simulink model "F28379D_benchTest_demo1_CPU1"  (R2019b)
settings: Solver=FixedStepDiscrete  StartTime=0.0  StopTime=Inf  RelTol=1e-3  EnableMultiTasking=on
PreLoadFcn:
  | RTWConfigurationCB('preloadfcn', bdroot);
undefined symbols (not defined in the file or in its folder): Down, GPTRIP1SEL, GPTRIP2SEL, LEDPWM, TZ1, TZ2, Up
libraries: c280xlib x3, simulink x3, c2837xDlib x3, c2802xlib x2, canmsglib x1, hdlsllib x1
settings Model: DataDictionary=F28379D_benchTest_demo1.sldd  ExtModeTrigDuration=8  Creator=Nick  LastModifiedBy=Nick
settings OptimizationCC: DefaultUnderspecifiedDataType=single  EnhancedBackFolding=on  PassReuseOutputArgsAs=Individual arguments  MaxStackSize=1024  OptimizeBlockOrder=speed  DifferentSizesBufferReuse=on  OptimizationCustomize=off  DenormalBehavior=FlushToZero  EfficientTunableParamExpr=on
settings DebuggingCC: ParameterTunabilityLossMsg=error
settings HardwareCC: ProdBitPerChar=16  ProdBitPerInt=16  ProdBitPerPointer=32  ProdBitPerSizeT=32  ProdBitPerPtrDiffT=32  ProdLargestAtomicInteger=Integer  ProdLargestAtomicFloat=None  ProdWordSize=16  ProdLongLongMode=on  ProdHWDeviceType=Texas Instruments->C2000
settings SFSimCC: MATLABDynamicMemAlloc=off
settings RTWCC: SystemTargetFile=ert.tlc  HardwareBoard=TI Delfino F28379D LaunchPad  TLCOptions=-aInlineSetEventsForThisBaseRateFcn=TLC_FALSE -aSuppressMultiTaskScheduler=TLC_FALSE -aRateBasedStepFcn=1  TemplateMakefile=ert_default_tmf  GenerateReport=on  Toolchain=Texas Instruments Code Composer Studio (C2000)  IncludeHyperlinkInReport=on  LaunchReport=on  GenerateTraceInfo=on  GenerateTraceReport=on  GenerateTraceReportSl=on  GenerateTraceReportSf=on  GenerateTraceReportEml=on
settings CodeAppCC: ForceParamTrailComments=on  IgnoreCustomStorageClasses=off  OperatorAnnotations=on  SimulinkDataObjDesc=on  SFDataObjDesc=on  InsertBlockDesc=on
settings ERTTargetCC: CodeReplacementLibrary=TI C28x  GenerateASAP2=on  ExtModeStaticAllocSize=10000

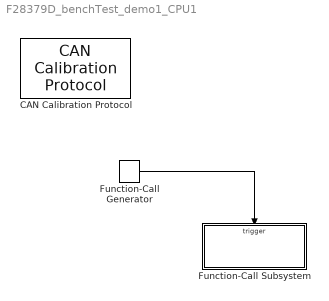
== system F28379D_benchTest_demo1_CPU1 ==
  CAN Calibration Protocol : c280xlib/CAN Calibration Protocol  CCP_STATION_ID=hex2dec('1')  module=eCAN_B  ccp_cro_id=hex2dec('6FA')  ccp_cro_message_type=Standard (11-bit identifier)  ccp_return_id=hex2dec('6FB')  ccp_return_message_type=Standard (11-bit identifier)  TOTAL_NUM_ODTS=20  cro_sample_time=0.1
      settings: SourceProductName=Embedded Coder Support Package for Texas Instruments C2000 Processors  SourceProductBaseCode=TIC2000
  Function-Call Generator : simulink/Ports & Subsystems/Function-Call Generator  sample_time=.001  numberOfIterations=1
  Function-Call Subsystem : Subsystem  TreatAsAtomicUnit=on
  wires:
  Function-Call Generator/1 -> Function-Call Subsystem/Trigger

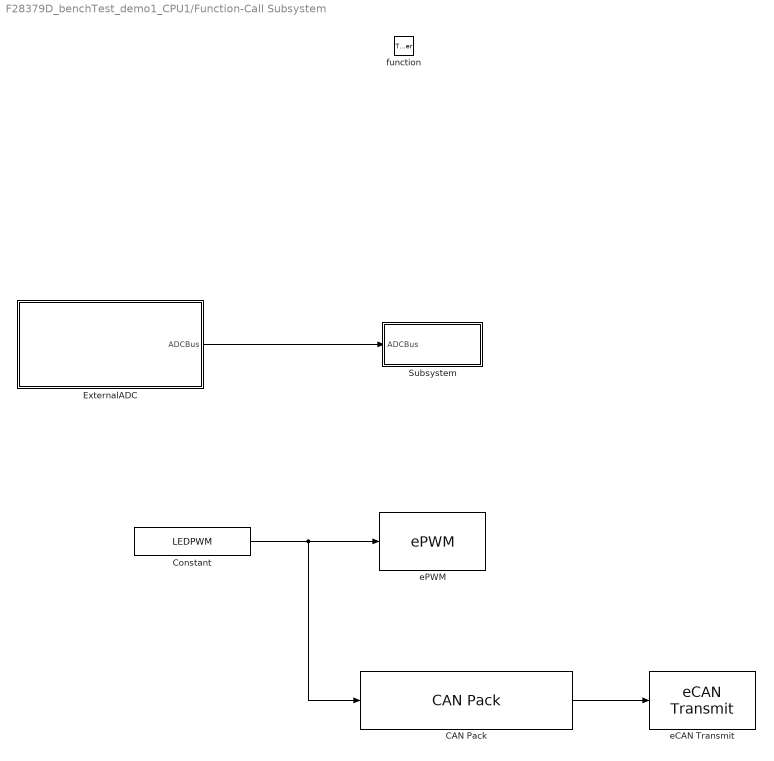
== system F28379D_benchTest_demo1_CPU1/Function-Call Subsystem ==
  function : TriggerPort  TriggerType=function-call  VariantControl=Variant
  CAN Pack : canmsglib/CAN Pack  MsgList=(none)  MsgName=CAN Msg  MsgIDType=Standard (11-bit identifier)  MsgIdentifier=10  MsgLength=8  Remote=off  ApplyMinMax=off  BusOutput=off  SignalInfo={ 'PWM', '0', '16', 'LE', 'signed', 'Standard', '0', '1', '0', '-Inf', 'Inf' }
      settings: SourceProductName=Vehicle Network Toolbox  SourceProductBaseCode=VN  DataFormat=manually specified signals
  Constant : Constant  Value=LEDPWM  SampleTime=-1
  ExternalADC : Subsystem
  Subsystem : Subsystem
  eCAN Transmit : c280xlib/eCAN Transmit  chipFamily=C280x  useModule=eCAN_B  mailboxNo=3  messageID=bin2dec('111000111')  messageType=Standard (11-bit identifier)  enableBlockingMode=off  postInterrupt=off  interruptLine=0
      settings: SourceProductName=Embedded Coder Support Package for Texas Instruments C2000 Processors  SourceProductBaseCode=TIC2000
  ePWM : c2802xlib/ePWM  useModule=ePWM12  ePWMxLINKTBPRD=Not Linked  periodUnits=Seconds  timerSource=Specify via dialog  timerPeriod_clk=64000  timerPeriod_sec=0.0001  tbshadow=Counter equals to zero  countingMode=Up-Down  phaseActiveEnable=Disable  phaseDirection=Count down after sync  phaseActive=0  synchronizationEnable=off  dcaevt1Sync=off  dcbevt1Sync=off  synchronizationOption=Disable  clockPrescale=1  HSclockPrescale=1  enswap=off  ePWMxAStatus=on  ePWMxAactionLogic1=Set  ePWMxAactionLogic2=Clear  ePWMxAactionLogic3=Clear  ePWMxAactionLogic4=Set  ePWMxAactionLogic5=Do nothing  ePWMxAactionLogic6=Do nothing  ePWMxALoadMode=Load on counter equals to zero (CTR=Zero)  ePWMxACSFenable=off  ePWMxACSFvalue=Forcing disable  ePWMxASFreload=Zero  ePWMxBStatus=off  ePWMxBactionLogic1=Set  ePWMxBactionLogic2=Clear  ePWMxBactionLogic3=Do nothing  ePWMxBactionLogic4=Do nothing  ePWMxBactionLogic5=Clear  ePWMxBactionLogic6=Set  ePWMxBLoadMode=Load on counter equals to zero (CTR=Zero)  ePWMxBCSFenable=off  ePWMxBCSFvalue=Forcing disable  ePWMxBSFreload=Zero  ePWNxBOutWay=off  ePWMxLINKCMPA=Not Linked  CMPAUnits=Percentages  CMPASource=Input port  CMPAValue_per=0  CMPAValue_clk=32000  enCMPAshadow=Counter equals to zero  ePWMxLINKCMPB=Not Linked  CMPBUnits=Clock cycles  CMPBSource=Specify via dialog  CMPBValue_per=50  CMPBValue_clk=32000  enCMPBshadow=Counter equals to zero  ePWMxLINKCMPC=Not Linked  CMPCUnits=Clock cycles  CMPCSource=Specify via dialog  CMPCValue_per=50  CMPCValue_clk=32000  enCMPCshadow=Counter equals to zero  ePWMxLINKCMPD=Not Linked  CMPDUnits=Clock cycles  CMPDSource=Specify via dialog  CMPDValue_per=50  CMPDValue_clk=32000  enCMPDshadow=Counter equals to zero  enableDBePWMxA=off  enableDBePWMxB=off  enhalfcycle=off  DBpolarity=Active high (AH)  DBedgeDelay=Positive  DBSource_ePWMxA=ePWMxA  DBSource_ePWMxB=ePWMxA  DBperiodSource=Specify via dialog  REDperiod=0  FEDperiod=0  adcstartModuleA=off  adcrequestEventA=First event  adcstartEventA=Digital Compare Module A Event 1 start of conversion (DCAEVT1.soc)  adcstartEventA_type2=Digital Compare Module A Event 1 start of conversion (DCAEVT1.soc)  adcstartModuleB=off  adcrequestEventB=First event  adcstartEventB=Counter equals to zero (CTR=Zero)  adcstartEventB_type2=Counter equals to zero (CTR=Zero)  intEn=off  intPrd=First event  intSel=Counter equals to zero (CTR=Zero)  intSel_type2=Counter equals to zero (CTR=Zero)  hrpe=off  enHRPWM=off  HRPWM_LoadMode=Counter equals to period (CTR=PRD)  HRPWM_CTLMode=Duty or Period control mode  HRPWM_EDGMode=Both edge  hrpeb=off  enHRPWMB=off  HRPWM_LoadModeB=Counter equals to zero (CTR=ZERO)  HRPWM_CTLModeB=Duty or Period control mode  HRPWM_EDGModeB=Both edge  enSFO=on  enautoconv=on  chopperEnable=off  chopperFrequency=1  chopperFirstwidth=1  chopperDuty=12.5%  tripZonesource=Specify via dialog  tzselOSHT1=off  tzselOSHT2=off  tzselOSHT3=off  tzselOSHDCAEV1=off  tzselOSHDCBEV1=off  tzselCBC1=off  tzselCBC2=off  tzselCBC3=off  tzselCBCDCAEV2=off  tzselCBCDCBEV2=off  tzselOSHT4=off  tzselOSHT5=off  tzselOSHT6=off  tzselCBC4=off  tzselCBC5=off  tzselCBC6=off  enTzOstIntr=off  enTzCbcIntr=off  enTzDCAEVT1Intr=off  enTzDCAEVT2Intr=off  enTzDCBEVT1Intr=off  enTzDCBEVT2Intr=off  ePWMxAforced=No action  ePWMxBforced=No action  DCAEVT1forced=No action  DCBEVT1forced=No action  DCAEVT2forced=No action  DCBEVT2forced=No action  dcah=Trip Zone 1 input (TZ1)  dcal=Trip Zone 2 input (TZ2)  dcbh=Trip Zone 1 input (TZ1)  dcbl=Trip Zone 2 input (TZ2)  dcah_type2=GPTRIP1SEL/(TZ1)  dcal_type2=GPTRIP2SEL/(TZ2)  dcbh_type2=GPTRIP1SEL/(TZ1)  dcbl_type2=GPTRIP2SEL/(TZ2)  gendcaevt1=Event disabled  gendcaevt2=Event disabled  gendcbevt1=Event disabled  gendcbevt2=Event disabled  dcaevt1src=DCAEVT1 with sync  dcaevt2src=DCAEVT2 with sync  dcbevt1src=DCBEVT1 with sync  dcbevt2src=DCBEVT2 with sync  pulsesel=Counter equals to zero (CTR=Zero)  blankinv=off  blankoffset=0  blankwidth=0  evsrcsel=Filtered version of DCAEVT1 (DCAEVT1FILT)  encape=off  PwmType=C2000_Type4
      settings: SourceProductName=Embedded Coder Support Package for Texas Instruments C2000 Processors
  wires:
  ExternalADC/1(ADCBus) -> Subsystem/1(ADCBus)
  Constant/1 -> CAN Pack/1, ePWM/1
  CAN Pack/1 -> eCAN Transmit/1

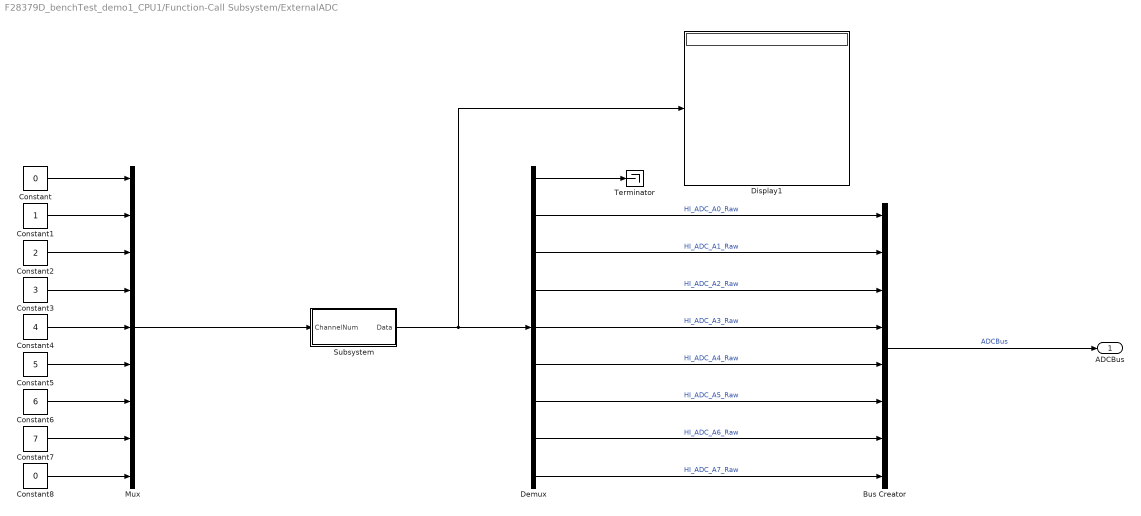
== system F28379D_benchTest_demo1_CPU1/Function-Call Subsystem/ExternalADC ==
  Bus Creator : BusCreator  Inputs=8
  Constant : Constant  Value=0
  Constant1 : Constant
  Constant2 : Constant  Value=2
  Constant3 : Constant  Value=3
  Constant4 : Constant  Value=4
  Constant5 : Constant  Value=5
  Constant6 : Constant  Value=6
  Constant7 : Constant  Value=7
  Constant8 : Constant  Value=0
  Demux : Demux  Outputs=9
  Display1 : Display
  Mux : Mux  Inputs=9
  Subsystem : Subsystem
  Terminator : Terminator
  ADCBus : Outport
  wires:
  Constant6/1 -> Mux/7
  Demux/1 -> Terminator/1
  Constant7/1 -> Mux/8
  Mux/1 -> Subsystem/1(ChannelNum)
  Demux/5 -> Bus Creator/4  "HI_ADC_A3_Raw"
  Constant8/1 -> Mux/9
  Demux/2 -> Bus Creator/1  "HI_ADC_A0_Raw"
  Constant2/1 -> Mux/3
  Demux/8 -> Bus Creator/7  "HI_ADC_A6_Raw"
  Demux/7 -> Bus Creator/6  "HI_ADC_A5_Raw"
  Constant5/1 -> Mux/6
  Constant/1 -> Mux/1
  Constant4/1 -> Mux/5
  Bus Creator/1 -> ADCBus/1  "ADCBus"
  Demux/3 -> Bus Creator/2  "HI_ADC_A1_Raw"
  Demux/9 -> Bus Creator/8  "HI_ADC_A7_Raw"
  Demux/4 -> Bus Creator/3  "HI_ADC_A2_Raw"
  Constant1/1 -> Mux/2
  Constant3/1 -> Mux/4
  Demux/6 -> Bus Creator/5  "HI_ADC_A4_Raw"
  Subsystem/1(Data) -> Display1/1, Demux/1

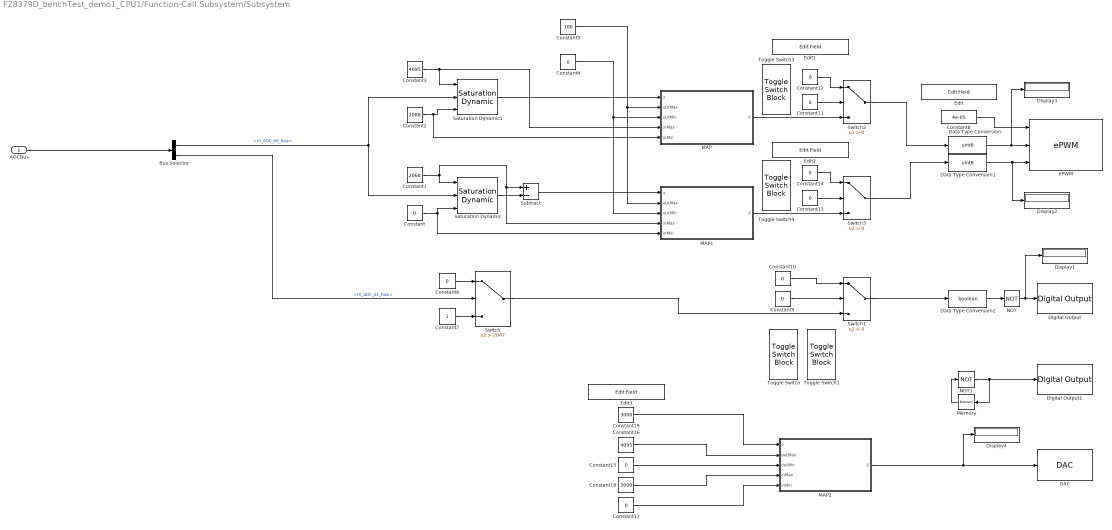
== system F28379D_benchTest_demo1_CPU1/Function-Call Subsystem/Subsystem ==
  ADCBus : Inport
  Bus Selector : BusSelector  OutputSignals=HI_ADC_A0_Raw,HI_ADC_A1_Raw
  Constant{,4,6,9..15,17} (11 alike) : Constant  Value=0
  Constant1 : Constant  Value=2068
  Constant16 : Constant  Value=4095
  Constant18 : Constant  Value=3000
  Constant19 : Constant  Value=3000
  Constant2 : Constant  Value=2088
  Constant3 : Constant  Value=4095
  Constant5 : Constant  Value=100
  Constant7 : Constant
  Constant8 : Constant  Value=4e-05
  DAC : c2837xDlib/DAC  channel=A  saturate=on
      settings: SourceProductName=Embedded Coder Support Package for Texas Instruments C2000 Processors  SourceProductBaseCode=TIC2000
  Data Type Conversion : DataTypeConversion  OutDataTypeStr=uint8
  Data Type Conversion1 : DataTypeConversion  OutDataTypeStr=uint8
  Data Type Conversion2 : DataTypeConversion  OutDataTypeStr=boolean
  Digital Output : c2837xDlib/Digital Output  GPIO_Number=GPIO16~GPIO23  GPIO_Bit0=on  GPIO_BIT0_Toggle=off  GPIO_Bit1=off  GPIO_BIT1_Toggle=off  GPIO_Bit2=off  GPIO_BIT2_Toggle=off  GPIO_Bit3=off  GPIO_BIT3_Toggle=off  GPIO_Bit4=off  GPIO_BIT4_Toggle=off  GPIO_Bit5=off  GPIO_BIT5_Toggle=off  GPIO_Bit6=off  GPIO_BIT6_Toggle=off  GPIO_Bit7=off  GPIO_BIT7_Toggle=off
      settings: SourceProductName=Embedded Coder Support Package for Texas Instruments C2000 Processors  SourceProductBaseCode=TIC2000
  Digital Output1 : c2837xDlib/Digital Output  GPIO_Number=GPIO64~GPIO71  GPIO_Bit0=off  GPIO_BIT0_Toggle=off  GPIO_Bit1=off  GPIO_BIT1_Toggle=off  GPIO_Bit2=off  GPIO_BIT2_Toggle=off  GPIO_Bit3=on  GPIO_BIT3_Toggle=off  GPIO_Bit4=off  GPIO_BIT4_Toggle=off  GPIO_Bit5=off  GPIO_BIT5_Toggle=off  GPIO_Bit6=off  GPIO_BIT6_Toggle=off  GPIO_Bit7=off  GPIO_BIT7_Toggle=off
      settings: SourceProductName=Embedded Coder Support Package for Texas Instruments C2000 Processors  SourceProductBaseCode=TIC2000
  Display{1..4} (4 alike) : Display
  Edit{,1..3} (4 alike) : EditField  LabelPosition=Hide  ShowInitialText=on  Alignment=Center
  MAP : Subsystem
  MAP1 : Subsystem
  MAP2 : Subsystem
  Memory : Memory  InheritSampleTime=on
  NOT : Logic  Operator=NOT  IconShape=distinctive  AllPortsSameDT=off  OutDataTypeStr=boolean
  NOT1 : Logic  Operator=NOT  IconShape=distinctive  AllPortsSameDT=off  OutDataTypeStr=boolean
  Saturation Dynamic : simulink/Discontinuities/Saturation Dynamic  OutMin=[]  OutMax=[]  OutDataTypeStr=Inherit: Same as second input  OutDataType=fixdt(1, 16)  OutScaling=2^-10  DoSatur=off
  Saturation Dynamic1 : simulink/Discontinuities/Saturation Dynamic  OutMin=[]  OutMax=[]  OutDataTypeStr=Inherit: Same as second input  OutDataType=fixdt(1, 16)  OutScaling=2^-10  DoSatur=off
  Subtract : Sum  Inputs=+-
  Switch : Switch  Criteria=u2 > Threshold  Threshold=2047
  Switch1 : Switch  Criteria=u2 > Threshold
  Switch2 : Switch  Criteria=u2 > Threshold
  Switch3 : Switch  Criteria=u2 > Threshold
  Toggle Switch{,1,3..4} (4 alike) : ToggleSwitchBlock
  ePWM : c2802xlib/ePWM  useModule=ePWM2  ePWMxLINKTBPRD=Not Linked  periodUnits=Seconds  timerSource=Input port  timerPeriod_clk=64000  timerPeriod_sec=0.0001  tbshadow=Counter equals to zero  countingMode=Up-Down  phaseActiveEnable=Disable  phaseDirection=Count down after sync  phaseActive=0  synchronizationEnable=off  dcaevt1Sync=off  dcbevt1Sync=off  synchronizationOption=Disable  clockPrescale=1  HSclockPrescale=1  enswap=off  ePWMxAStatus=on  ePWMxAactionLogic1=Set  ePWMxAactionLogic2=Clear  ePWMxAactionLogic3=Clear  ePWMxAactionLogic4=Set  ePWMxAactionLogic5=Do nothing  ePWMxAactionLogic6=Do nothing  ePWMxALoadMode=Load on counter equals to zero (CTR=Zero)  ePWMxACSFenable=off  ePWMxACSFvalue=Forcing disable  ePWMxASFreload=Zero  ePWMxBStatus=on  ePWMxBactionLogic1=Set  ePWMxBactionLogic2=Clear  ePWMxBactionLogic3=Do nothing  ePWMxBactionLogic4=Do nothing  ePWMxBactionLogic5=Clear  ePWMxBactionLogic6=Set  ePWMxBLoadMode=Load on counter equals to zero (CTR=Zero)  ePWMxBCSFenable=off  ePWMxBCSFvalue=Forcing disable  ePWMxBSFreload=Zero  ePWNxBOutWay=off  ePWMxLINKCMPA=Not Linked  CMPAUnits=Percentages  CMPASource=Input port  CMPAValue_per=0  CMPAValue_clk=32000  enCMPAshadow=Counter equals to zero  ePWMxLINKCMPB=Not Linked  CMPBUnits=Percentages  CMPBSource=Input port  CMPBValue_per=0  CMPBValue_clk=32000  enCMPBshadow=Counter equals to zero  ePWMxLINKCMPC=Not Linked  CMPCUnits=Clock cycles  CMPCSource=Specify via dialog  CMPCValue_per=50  CMPCValue_clk=32000  enCMPCshadow=Counter equals to zero  ePWMxLINKCMPD=Not Linked  CMPDUnits=Clock cycles  CMPDSource=Specify via dialog  CMPDValue_per=50  CMPDValue_clk=32000  enCMPDshadow=Counter equals to zero  enableDBePWMxA=off  enableDBePWMxB=off  enhalfcycle=off  DBpolarity=Active high (AH)  DBedgeDelay=Positive  DBSource_ePWMxA=ePWMxA  DBSource_ePWMxB=ePWMxA  DBperiodSource=Specify via dialog  REDperiod=0  FEDperiod=0  adcstartModuleA=off  adcrequestEventA=First event  adcstartEventA=Digital Compare Module A Event 1 start of conversion (DCAEVT1.soc)  adcstartEventA_type2=Digital Compare Module A Event 1 start of conversion (DCAEVT1.soc)  adcstartModuleB=off  adcrequestEventB=First event  adcstartEventB=Counter equals to zero (CTR=Zero)  adcstartEventB_type2=Counter equals to zero (CTR=Zero)  intEn=off  intPrd=First event  intSel=Counter equals to zero (CTR=Zero)  intSel_type2=Counter equals to zero (CTR=Zero)  hrpe=off  enHRPWM=off  HRPWM_LoadMode=Counter equals to period (CTR=PRD)  HRPWM_CTLMode=Duty or Period control mode  HRPWM_EDGMode=Both edge  hrpeb=off  enHRPWMB=off  HRPWM_LoadModeB=Counter equals to zero (CTR=ZERO)  HRPWM_CTLModeB=Duty or Period control mode  HRPWM_EDGModeB=Both edge  enSFO=on  enautoconv=on  chopperEnable=off  chopperFrequency=1  chopperFirstwidth=1  chopperDuty=12.5%  tripZonesource=Specify via dialog  tzselOSHT1=off  tzselOSHT2=off  tzselOSHT3=off  tzselOSHDCAEV1=off  tzselOSHDCBEV1=off  tzselCBC1=off  tzselCBC2=off  tzselCBC3=off  tzselCBCDCAEV2=off  tzselCBCDCBEV2=off  tzselOSHT4=off  tzselOSHT5=off  tzselOSHT6=off  tzselCBC4=off  tzselCBC5=off  tzselCBC6=off  enTzOstIntr=off  enTzCbcIntr=off  enTzDCAEVT1Intr=off  enTzDCAEVT2Intr=off  enTzDCBEVT1Intr=off  enTzDCBEVT2Intr=off  ePWMxAforced=No action  ePWMxBforced=No action  DCAEVT1forced=No action  DCBEVT1forced=No action  DCAEVT2forced=No action  DCBEVT2forced=No action  dcah=Trip Zone 1 input (TZ1)  dcal=Trip Zone 2 input (TZ2)  dcbh=Trip Zone 1 input (TZ1)  dcbl=Trip Zone 2 input (TZ2)  dcah_type2=GPTRIP1SEL/(TZ1)  dcal_type2=GPTRIP2SEL/(TZ2)  dcbh_type2=GPTRIP1SEL/(TZ1)  dcbl_type2=GPTRIP2SEL/(TZ2)  gendcaevt1=Event disabled  gendcaevt2=Event disabled  gendcbevt1=Event disabled  gendcbevt2=Event disabled  dcaevt1src=DCAEVT1 with sync  dcaevt2src=DCAEVT2 with sync  dcbevt1src=DCBEVT1 with sync  dcbevt2src=DCBEVT2 with sync  pulsesel=Counter equals to zero (CTR=Zero)  blankinv=off  blankoffset=0  blankwidth=0  evsrcsel=Filtered version of DCAEVT1 (DCAEVT1FILT)  encape=off  PwmType=C2000_Type4
      settings: SourceProductName=Embedded Coder Support Package for Texas Instruments C2000 Processors
  wires:
  ADCBus/1 -> Bus Selector/1
  Bus Selector/1 -> Saturation Dynamic/2, Saturation Dynamic1/2  "<HI_ADC_A0_Raw>"
  Constant/1 -> MAP1/5(inMin), Saturation Dynamic/3
  Constant1/1 -> Subtract/1, MAP1/4(inMax), Saturation Dynamic/1
  Subtract/1 -> MAP1/1(x)
  Constant3/1 -> Saturation Dynamic1/1, MAP/4(inMax)
  Constant2/1 -> MAP/5(inMin), Saturation Dynamic1/3
  Saturation Dynamic1/1 -> MAP/1(x)
  Constant4/1 -> MAP1/3(outMin), MAP/3(outMin)
  Constant5/1 -> MAP1/2(outMax), MAP/2(outMax)
  MAP/1(X) -> Switch2/3
  Saturation Dynamic/1 -> Subtract/2
  Switch/1 -> Switch1/3
  Bus Selector/2 -> Switch/2  "<HI_ADC_A1_Raw>"
  Constant6/1 -> Switch/1
  Constant7/1 -> Switch/3
  Data Type Conversion/1 -> Display3/1, ePWM/2
  Data Type Conversion1/1 -> Display2/1, ePWM/3
  Constant8/1 -> ePWM/1
  Data Type Conversion2/1 -> NOT/1
  NOT/1 -> Display1/1, Digital Output/1
  Switch1/1 -> Data Type Conversion2/1
  Constant9/1 -> Switch1/2
  Constant10/1 -> Switch1/1
  Switch2/1 -> Data Type Conversion/1
  Constant11/1 -> Switch2/2
  Constant12/1 -> Switch2/1
  Switch3/1 -> Data Type Conversion1/1
  MAP1/1(X) -> Switch3/3
  Constant13/1 -> Switch3/2
  Constant14/1 -> Switch3/1
  Memory/1 -> NOT1/1
  NOT1/1 -> Memory/1, Digital Output1/1
  MAP2/1(X) -> Display4/1, DAC/1
  Constant16/1 -> MAP2/2(outMax)
  Constant15/1 -> MAP2/3(outMin)
  Constant18/1 -> MAP2/4(inMax)
  Constant17/1 -> MAP2/5(inMin)
  Constant19/1 -> MAP2/1(x)

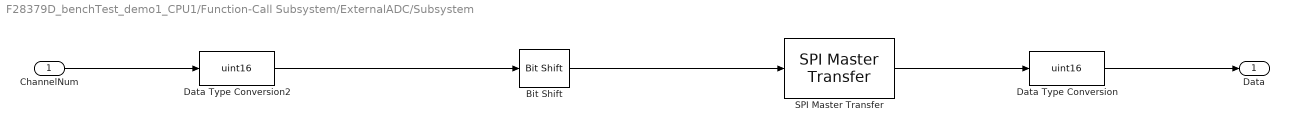
== system F28379D_benchTest_demo1_CPU1/Function-Call Subsystem/ExternalADC/Subsystem ==
  ChannelNum : Inport
  Bit Shift : hdlsllib/Logic and Bit Operations/Bit Shift  mode=Shift Left Logical  N=11
      settings: SourceProductName=Simulink
  Data Type Conversion : DataTypeConversion  OutDataTypeStr=uint16
  Data Type Conversion2 : DataTypeConversion  OutDataTypeStr=uint16
  SPI Master Transfer : c280xlib/SPI Master Transfer  SPISelect=SPI_A  ClockPolarity=Falling_edge  ClockPhase=No_delay  SPIModule=uint32(0)  Mode=Master  BusSpeed=uint32(1000000)  FirstBitToTransfer=Most significant bit (MSB)  ClockMode=0  BlockFunction=Transfer  EnableRegisterAddress=on  RegisterAddress=0  OutputDataType=int8  OutputDataLength=1  DataBits=16  UseCustomSSPin=Explicit GPIO calls  ActiveLowSSPin=Active low  Pin=19
      settings: SourceProductName=Embedded Coder Support Package for Texas Instruments C2000 Processors  SourceProductBaseCode=TIC2000
  Data : Outport
  wires:
  ChannelNum/1 -> Data Type Conversion2/1
  Data Type Conversion/1 -> Data/1
  SPI Master Transfer/1 -> Data Type Conversion/1
  Data Type Conversion2/1 -> Bit Shift/1
  Bit Shift/1 -> SPI Master Transfer/1

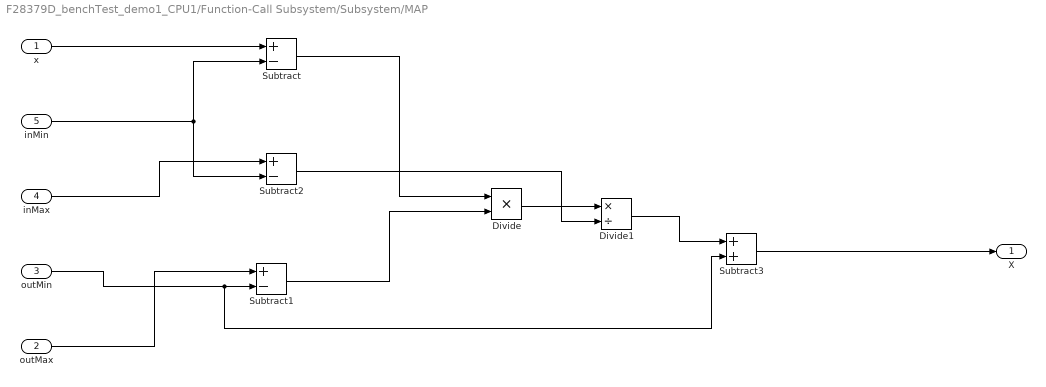
== system F28379D_benchTest_demo1_CPU1/Function-Call Subsystem/Subsystem/MAP ==
  x : Inport
  outMax : Inport  Port=2
  outMin : Inport  Port=3
  inMax : Inport  Port=4
  inMin : Inport  Port=5
  Divide : Product  Inputs=**
  Divide1 : Product  Inputs=*/
  Subtract : Sum  Inputs=+-
  Subtract1 : Sum  Inputs=+-
  Subtract2 : Sum  Inputs=+-
  Subtract3 : Sum
  X : Outport
  wires:
  x/1 -> Subtract/1
  inMin/1 -> Subtract2/2, Subtract/2
  Subtract/1 -> Divide/1
  outMax/1 -> Subtract1/1
  outMin/1 -> Subtract3/2, Subtract1/2
  Subtract1/1 -> Divide/2
  inMax/1 -> Subtract2/1
  Subtract2/1 -> Divide1/2
  Divide/1 -> Divide1/1
  Divide1/1 -> Subtract3/1
  Subtract3/1 -> X/1

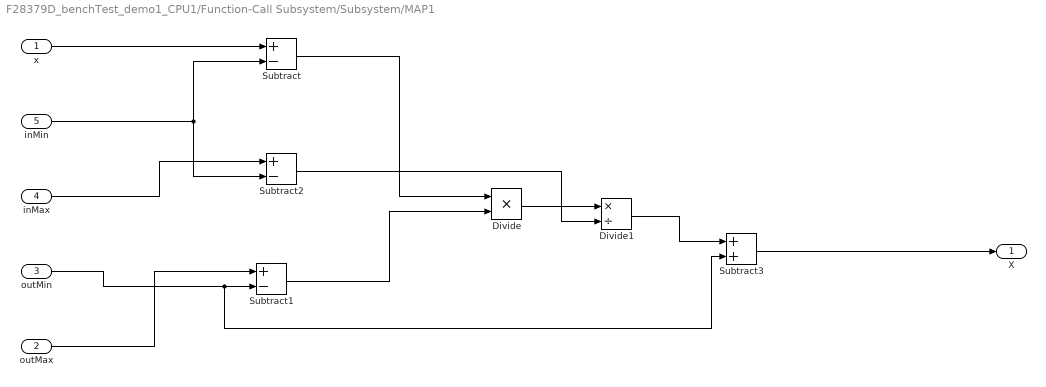
== system F28379D_benchTest_demo1_CPU1/Function-Call Subsystem/Subsystem/MAP1 ==
  x : Inport
  outMax : Inport  Port=2
  outMin : Inport  Port=3
  inMax : Inport  Port=4
  inMin : Inport  Port=5
  Divide : Product  Inputs=**
  Divide1 : Product  Inputs=*/
  Subtract : Sum  Inputs=+-
  Subtract1 : Sum  Inputs=+-
  Subtract2 : Sum  Inputs=+-
  Subtract3 : Sum
  X : Outport
  wires:
  x/1 -> Subtract/1
  inMin/1 -> Subtract2/2, Subtract/2
  Subtract/1 -> Divide/1
  outMax/1 -> Subtract1/1
  outMin/1 -> Subtract3/2, Subtract1/2
  Subtract1/1 -> Divide/2
  inMax/1 -> Subtract2/1
  Subtract2/1 -> Divide1/2
  Divide/1 -> Divide1/1
  Divide1/1 -> Subtract3/1
  Subtract3/1 -> X/1

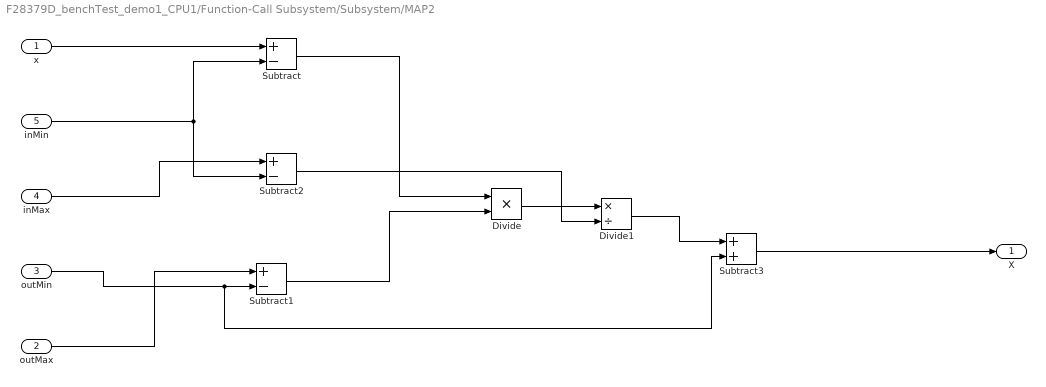
== system F28379D_benchTest_demo1_CPU1/Function-Call Subsystem/Subsystem/MAP2 ==
  x : Inport
  outMax : Inport  Port=2
  outMin : Inport  Port=3
  inMax : Inport  Port=4
  inMin : Inport  Port=5
  Divide : Product  Inputs=**
  Divide1 : Product  Inputs=*/
  Subtract : Sum  Inputs=+-
  Subtract1 : Sum  Inputs=+-
  Subtract2 : Sum  Inputs=+-
  Subtract3 : Sum
  X : Outport
  wires:
  x/1 -> Subtract/1
  inMin/1 -> Subtract2/2, Subtract/2
  Subtract/1 -> Divide/1
  outMax/1 -> Subtract1/1
  outMin/1 -> Subtract3/2, Subtract1/2
  Subtract1/1 -> Divide/2
  inMax/1 -> Subtract2/1
  Subtract2/1 -> Divide1/2
  Divide/1 -> Divide1/1
  Divide1/1 -> Subtract3/1
  Subtract3/1 -> X/1
